simulink model "ORGANIZED_NominalTracking"  (R2024b)
settings: Solver=ode45  StartTime=0.0  StopTime=10  RelTol=1e-3
values from neighbouring files (symbols this model uses):
  current2Torque = mot.Kt    [simulation.m]
  denDriv = [Tdrv 1]    [simulation.m]
  denElect = [mot.L Req]    [simulation.m]
  denMech = [J_eq B_eq]    [simulation.m]
  numDriv = [kdrv]    [simulation.m]
  numElect = [1]    [simulation.m]
  numMech = [1]    [simulation.m]
  speed2Voltage = mot.Ke    [simulation.m]
undefined symbols (not defined in the file or in its folder): daq, degs2rpm, denBeam, denHPF, drv, gbox, kappa, mld, numBeam, numHPF, rads2rpm, rpm2rads, sens, ssc, ssc_LQR
settings Model: Creator=llp  LastModifiedBy=llp

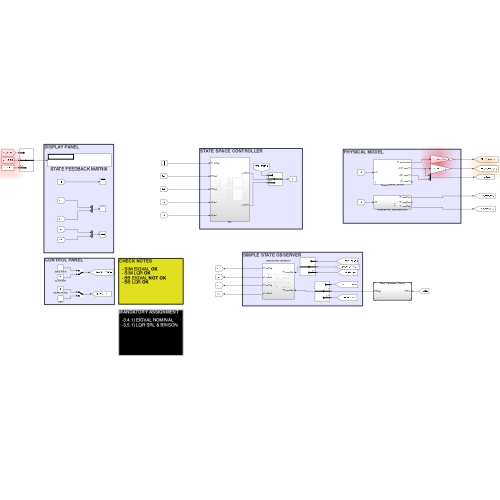
[thumbnail: Simulink's stored preview of the top-level diagram]
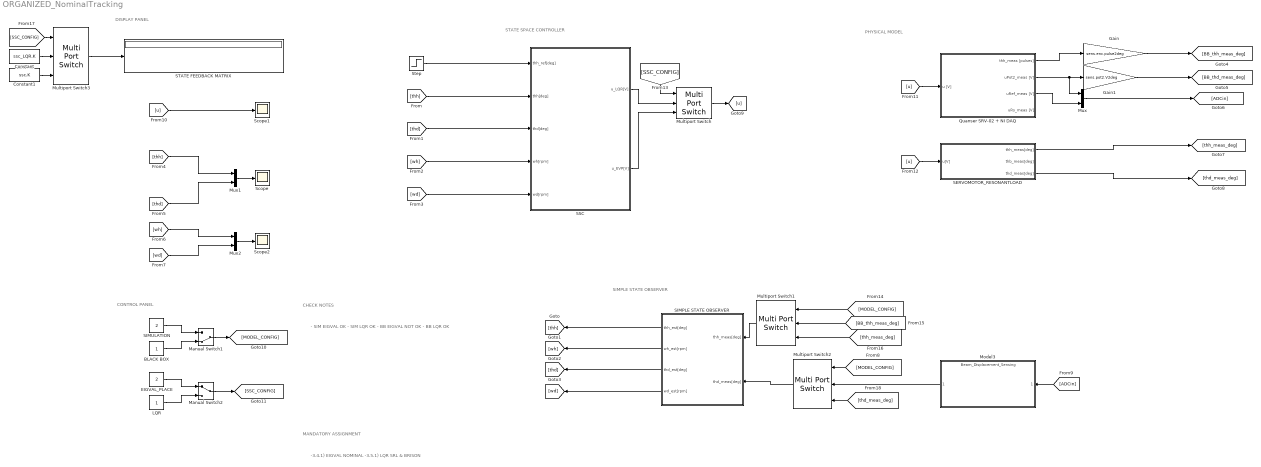
== system ORGANIZED_NominalTracking ==
  note: - SIM EIGVAL OK
      | - SIM LQR OK
      | - BB EIGVAL NOT OK
      | - BB LQR OK
  note: CHECK NOTES
  note: PHYSICAL MODEL
  note: STATE SPACE CONTROLLER
  note: SIMPLE STATE OBSERVER
  note: CONTROL PANEL
  note: DISPLAY PANEL
  note: -3.4.1) EIGVAL NOMINAL
      | -3.5.1) LQR SRL & BRISON
  note: MANDATORY ASSIGNMENT
  BLACK BOX : Constant
  Constant : Constant  Value=ssc_LQR.K
  Constant1 : Constant  Value=ssc.K
  EIGVAL_PLACE : Constant  Value=2
  Gain : Gain  Gain=sens.enc.pulse2deg
  Gain1 : Gain  Gain=sens.pot2.V2deg
  LQR : Constant
  Manual Switch1 : ManualSwitch  CurrentSetting=0
  Manual Switch2 : ManualSwitch
  Model3 : ModelReference  ModelNameDialog=Beam_Displacement_Sensing.slx  SimulationMode=Normal  ModelReferenceVersion=1.3
  Multiport Switch{,1..3} (4 alike) : MultiPortSwitch  Inputs=2  SaturateOnIntegerOverflow=off  InputSameDT=off
  Mux : Mux  Inputs=2
  Mux1 : Mux  Inputs=2
  Mux2 : Mux  Inputs=2
  Quanser SRV-02 + NI DAQ : Subsystem  mask(Quanser SRV-02 (with resonant load) + NI DAQ){Ts=0.001, fricType=Coulomb + viscous, lockShaft=off, beamInitPos=10}
      mask prompts: Ts "NI DAQ Sample Time:"; fricType "Friction model"; lockShaft "Lock motor shaft"; beamInitPos "Beam initial position [deg]:"
      mask help: Quanser SRV-02 (with resonant load) + NI DAQ model.
      mask init:
      | %%
      | % Riccardo Antonello (riccardo.antonello@unipd.it)
      | %
      | % April 28, 2020
      | %
      | % Dept. of Information Engineering, University of Padova
      | %
      | 
      | %%  Conversion gains
      | deg2rad = pi/180;                   %   [deg]   -> [rad]
      | rad2deg = 180/pi;                   %   [rad]   -> [deg]
      | 
      | 
      | %%  Sensors data
      | 
      | %   shunt resistor
      | sens.curr.Rs = 0.5;   
      | 
      | %   Hewlett-Packard HEDS-5540#A06 optical encoder
      | sens.enc.ppr = 500*4;                                                   %   pulses per rotation
      | sens.enc.pulse2deg = 360/sens.enc.ppr;                                  %   [pulses] -> [deg]
      | sens.enc.pulse2rad = 2*pi/sens.enc.ppr;                                 %   [pulses] -> [rad]
      | sens.enc.deg2pulse = sens.enc.ppr/360;                                  %   [deg] -> [pulses]
      | sens.enc.rad2pulse = sens.enc.ppr/2/pi;                                 %   [rad] -> [pulses]
      | 
      | %   potentiometer 2 (Spectrol 357-0-0-103) - installed on hub
      | sens.pot2.range.R      = 10e3;                                          %   ohmic value range 
      | sens.pot2.range.V      = 5;                                             %   voltage range
      | sens.pot2.range.th_deg = 340;                                           %   angle range [deg]
      | sens.pot2.range.th     = sens.pot2.range.th_deg * deg2rad;              %   angle range [rad]                           
      | sens.pot2.deg2V        = sens.pot2.range.V / sens.pot2.range.th_deg;    %   sensitivity [V/deg]
      | sens.pot2.rad2V        = sens.pot2.range.V / sens.pot2.range.th;        %   sensitivity [V/rad]
      | sens.pot2.V2deg        = 1/sens.pot2.deg2V;                             %   conversion gain [V] -> [deg]
      | sens.pot2.V2rad        = 1/sens.pot2.rad2V;                             %   conversion gain [V] -> [rad]
      | sens.pot2.noise.var    = 3.5e-7;                                        %   out noise variance [V^2]
      | 
      | 
      | %%  Data acquisition board (daq) data
      | 
      | %   NI PCI-6221 DAC data
      | daq.dac.bits = 16;                                  %   resolution (bits)
      | daq.dac.fs   = 10;                                  %   full scale 
      | daq.dac.q    = 2*daq.dac.fs/(2^daq.dac.bits-1);     %	quantization
      | 
      | %   NI PCI-6221 ADC data
      | daq.adc.bits = 16;                                  %   resolution (bits)
      | daq.adc.fs   = 10;                                  %   full scale (as set in SLDRT Analog Input block)
      | daq.adc.q    = 2*daq.adc.fs/(2^daq.adc.bits-1);     %   quantization   
      | 
      | 
      | %%  Set beam initial position
      | % SRV02Handle = find_system(gcb, ...
      | %     'LookUnderMasks', 'on', ...
      | %     'FindAll', 'on', ...
      | %     'FollowLinks', 'on', ...
      | %     'SearchDepth', '1', ...
      | %     'BlockType', 'ModelReference', ...
      | %     'Name', 'Quanser SRV-02');
      | %
      | % %get_param(SRV02Handle, 'InstanceParameters')
      | % InstanceParams = get_param(SRV02Handle, 'InstanceParameters');
      | % for k = 1:length(InstanceParams)
      | %     if strcmp(InstanceParams(k).Name, 'thb0')
      | %         if lockShaft
      | %             InstanceParams(k).Value = sprintf('%f', beamInitPos);
      | %         else
      | %             InstanceParams(k).Value = sprintf('%f', 0);    
      | %         end
      | %         set_param(SRV02Handle, 'InstanceParameters', InstanceParams);
      | %         break;
      | %     end
      | % end
      | 
      | if lockShaft
      |     thb0 = beamInitPos;
      | else
      |     thb0 = 0;    
      | end
      | 
      | 
      | %%  Mask initialization
      | if lockShaft
      |     
      |     %   find Inport handle
      |     InPortHandle = find_system(gcb, ...
      |         'LookUnderMasks', 'on', ...
      |         'FindAll', 'on', ...
      |         'FollowLinks', 'on', ...
      |         'SearchDepth', '1', ...
      |         'BlockType', 'Inport', ...
      |         'Name', 'u [V]');
      |     
      |     if ~isempty(InPortHandle)
      |     
      |         %   find DAC handle
      |         DACHandle = find_system(gcb, ...
      |             'LookUnderMasks', 'on', ...
      |             'FindAll', 'on', ...
      |             'FollowLinks', 'on', ...
      |             'SearchDepth', '1', ...
      |             'BlockType', 'SubSystem', ...
      |             'Name', 'DAC');  
      | 
      |         %   remove Inport output connection   
      |         InportConn = get_param(InPortHandle, 'PortConnectivity');
      |         delete_line(gcb, InportConn.Position);
      | 
      |         %   remove Inport block
      |         delete_block(InPortHandle);
      | 
      |         %   add Constant block
      |         ConstantHandle = add_block( ...
      |             'simulink/Sources/Constant', [gcb, '/u [V]'], ...
      |             'Position', [20   -37    50   -23], ...
      |             'Value', '0');
      | 
      |         %   connect Constant to DAC block
      |         DACPortHandles = get_param(DACHandle, 'PortHandles');
      |         ConstantPortHandles = get_param(ConstantHandle, 'PortHandles');
      |         add_line(gcb, ConstantPortHandles.Outport(1), DACPortHandles.Inport(1));
      |     
      |     end
      |     
      | else
      |     
      |     %   find Constant handle
      |     ConstantHandle = find_system(gcb, ...
      |         'LookUnderMasks', 'on', ...
      |         'FindAll', 'on', ...
      |         'FollowLinks', 'on', ...
      |         'SearchDepth', '1', ...
      |         'BlockType', 'Constant', ...
      |         'Name', 'u [V]');
      |     
      |     if ~isempty(ConstantHandle)
      |     
      |         %   find DAC handle
      |         DACHandle = find_system(gcb, ...
      |             'LookUnderMasks', 'on', ...
      |             'FindAll', 'on', ...
      |             'FollowLinks', 'on', ...
      |             'SearchDepth', '1', ...
      |             'BlockType', 'SubSystem', ...
      |             'Name', 'DAC');  
      |  
      |         %   remove Constant output connection   
      |         ConstantConn = get_param(ConstantHandle, 'PortConnectivity');
      |         delete_line(gcb, ConstantConn.Position);
      | 
      |         %   remove Inport block
      |         delete_block(ConstantHandle);   
      | 
      |         %   add Inport block
      |         InportHandle = add_block( ...
      |             'simulink/Sources/In1', [gcb, '/u [V]'], ...
      |             'Position', [20   -37    50   -23], ...
      |             'Port', '1');
      | 
      |         %   connect Constant to DAC block
      |         DACPortHandles = get_param(DACHandle, 'PortHandles');
      |         InportPortHandles = get_param(InportHandle, 'PortHandles');
      |         add_line(gcb, InportPortHandles.Outport(1), DACPortHandles.Inport(1));
      |     
      |      end
      |     
      | end
      mask Help:
      | Riccardo Antonello (antonello@dei.unipd.it)
      | 
      | April 28, 2020
      | 
      | Dept. of Information Engineering, University of Padova
      mask TypeOptions fricType: Coulomb + viscous | Karnopp
      mask Callback lockShaft:
      | %   get status of check box
      | lockShaft = get_param(gcb, 'lockShaft');
      | 
      | %   get current value of MaskVisibilities property
      | maskVisibilities = get_param(gcb, 'MaskVisibilities');
      | 
      | %   set visibility of the dialog box element
      | if strcmp(lockShaft, 'on')
      |     maskVisibilities{4} = 'on';
      | else
      |     maskVisibilities{4} = 'off';
      | end
      | 
      | % Set the 'MaskVisibilities' property for each parameter in mask
      | set_param( gcb, 'MaskVisibilities', maskVisibilities);
  SERVOMOTOR_RESONANTLOAD : Subsystem
  SIMPLE STATE OBSERVER : Subsystem
  SIMULATION : Constant  Value=2
  SSC : Subsystem
  STATE FEEDBACK MATRIX : Display
  Scope : Scope
  Scope1 : Scope
  Scope2 : Scope
  Step : Step  After=0  SampleTime=0
  wires:
  SIMPLE STATE OBSERVER/2(wh_est[rpm]) -> [wh]
  [thd] -> SSC/3(thd[deg])
  Gain/1 -> [BB_thh_meas_deg]
  Quanser SRV-02 + NI DAQ/2(uPot2_meas [V]) -> Mux/1, Gain1/1
  SIMPLE STATE OBSERVER/4(wd_est[rpm]) -> [wd]
  [wd] -> Mux2/2
  Mux1/1 -> Scope/1
  [wh] -> Mux2/1
  [thh] -> Mux1/1
  Quanser SRV-02 + NI DAQ/1(thh_meas [pulses]) -> Gain/1
  Mux2/1 -> Scope2/1
  Quanser SRV-02 + NI DAQ/3(uRef_meas [V]) -> Mux/2
  SIMPLE STATE OBSERVER/1(thh_est[deg]) -> [thh]
  SIMPLE STATE OBSERVER/3(thd_est[deg]) -> [thd]
  [thd] -> Mux1/2
  [thh] -> SSC/2(thh[deg])
  Gain1/1 -> [BB_thd_meas_deg]
  Mux/1 -> [ADCin]
  [ADCin] -> Model3/1
  SERVOMOTOR_RESONANTLOAD/3(thd_meas[deg]) -> [thd_meas_deg]
  SERVOMOTOR_RESONANTLOAD/1(thh_meas[deg]) -> [thh_meas_deg]
  Multiport Switch/1 -> [u]
  [u] -> Scope1/1
  [u] -> SERVOMOTOR_RESONANTLOAD/1(u[V])
  [wd] -> SSC/5(wd[rpm])
  [wh] -> SSC/4(wh[rpm])
  Step/1 -> SSC/1(thh_ref[deg])
  SSC/1(u_LQR[V]) -> Multiport Switch/2
  Manual Switch1/1 -> [MODEL_CONFIG]
  SIMULATION/1 -> Manual Switch1/1
  BLACK BOX/1 -> Manual Switch1/2
  LQR/1 -> Manual Switch2/2
  Manual Switch2/1 -> [SSC_CONFIG]
  EIGVAL_PLACE/1 -> Manual Switch2/1
  [SSC_CONFIG] -> Multiport Switch/1
  SSC/2(u_EVP[V]) -> Multiport Switch/3
  [MODEL_CONFIG] -> Multiport Switch1/1
  [BB_thh_meas_deg] -> Multiport Switch1/2
  [thh_meas_deg] -> Multiport Switch1/3
  [MODEL_CONFIG] -> Multiport Switch2/1
  Model3/1 -> Multiport Switch2/2
  [thd_meas_deg] -> Multiport Switch2/3
  Multiport Switch2/1 -> SIMPLE STATE OBSERVER/2(thd_meas[deg])
  Multiport Switch1/1 -> SIMPLE STATE OBSERVER/1(thh_meas[deg])
  [SSC_CONFIG] -> Multiport Switch3/1
  Constant/1 -> Multiport Switch3/2
  Constant1/1 -> Multiport Switch3/3
  Multiport Switch3/1 -> STATE FEEDBACK MATRIX/1
  [u] -> Quanser SRV-02 + NI DAQ/1(u [V])

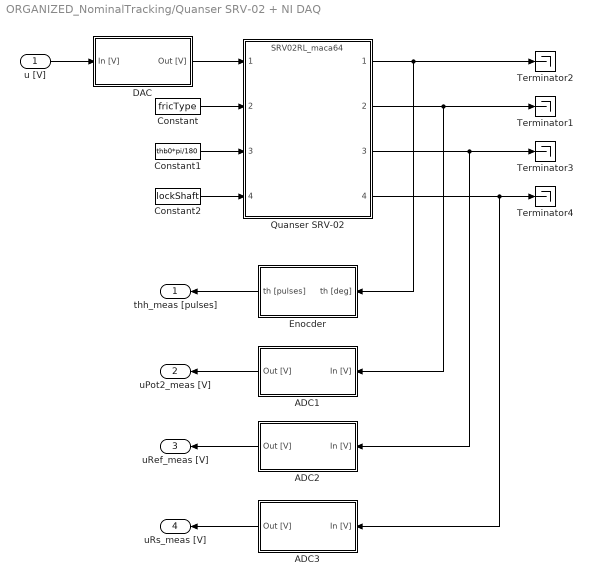
== system ORGANIZED_NominalTracking/Quanser SRV-02 + NI DAQ ==
  u [V] : Inport
  ADC1 : Subsystem
  ADC2 : Subsystem
  ADC3 : Subsystem
  Constant : Constant  Value=fricType
  Constant1 : Constant  Value=thb0*pi/180  SampleTime=Inf
  Constant2 : Constant  Value=lockShaft  SampleTime=Inf
  DAC : Subsystem
  Enocder : Subsystem
  Quanser SRV-02 : ModelReference  ModelNameDialog=SRV02RL_maca64.slxp  ModelReferenceVersion=1.76  CopyOfModelProtected=on
  Terminator{1..4} (4 alike) : Terminator
  thh_meas [pulses] : Outport
  uPot2_meas [V] : Outport  Port=2
  uRef_meas [V] : Outport  Port=3
  uRs_meas [V] : Outport  Port=4
  wires:
  Enocder/1(th [pulses]) -> thh_meas [pulses]/1
  ADC3/1(Out [V]) -> uRs_meas [V]/1
  DAC/1(Out [V]) -> Quanser SRV-02/1
  Quanser SRV-02/2 -> ADC1/1(In [V]), Terminator1/1
  Quanser SRV-02/1 -> Terminator2/1, Enocder/1(th [deg])
  Constant/1 -> Quanser SRV-02/2
  Quanser SRV-02/3 -> ADC2/1(In [V]), Terminator3/1
  ADC1/1(Out [V]) -> uPot2_meas [V]/1
  Constant1/1 -> Quanser SRV-02/3
  Constant2/1 -> Quanser SRV-02/4
  Quanser SRV-02/4 -> ADC3/1(In [V]), Terminator4/1
  ADC2/1(Out [V]) -> uRef_meas [V]/1
  u [V]/1 -> DAC/1(In [V])

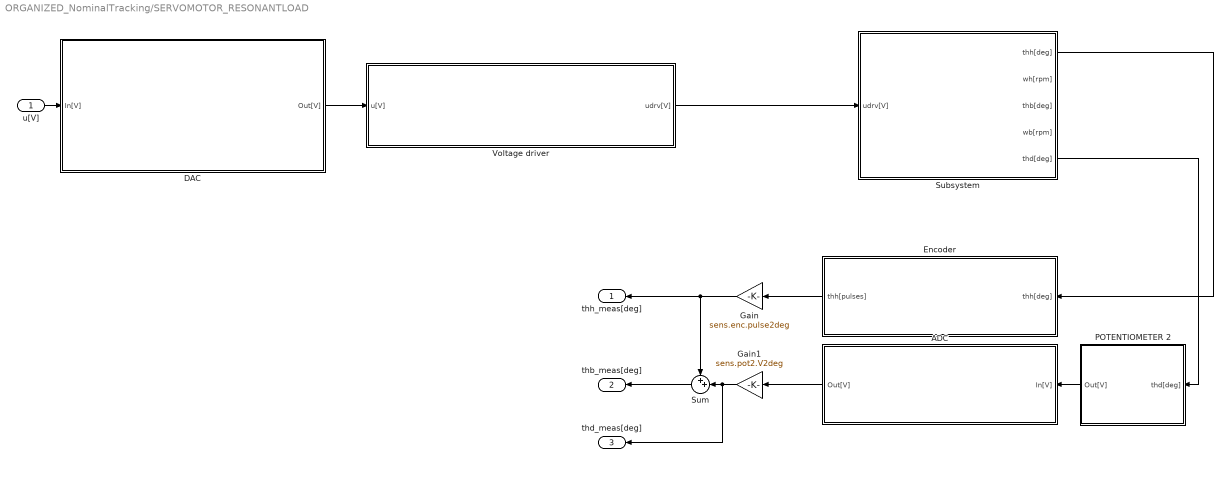
== system ORGANIZED_NominalTracking/SERVOMOTOR_RESONANTLOAD ==
  u[V] : Inport
  ADC : Subsystem
  DAC : Subsystem
  Encoder : Subsystem
  Gain : Gain  Gain=sens.enc.pulse2deg
  Gain1 : Gain  Gain=sens.pot2.V2deg
  POTENTIOMETER 2 : Subsystem
  Subsystem : Subsystem
  Sum : Sum  Inputs=++|
  Voltage driver : Subsystem
  thh_meas[deg] : Outport
  thb_meas[deg] : Outport  Port=2
  thd_meas[deg] : Outport  Port=3
  wires:
  Sum/1 -> thb_meas[deg]/1
  POTENTIOMETER 2/1(Out[V]) -> ADC/1(In[V])
  Gain/1 -> Sum/1, thh_meas[deg]/1
  ADC/1(Out[V]) -> Gain1/1
  u[V]/1 -> DAC/1(In[V])
  Encoder/1(thh[pulses]) -> Gain/1
  Subsystem/1(thh[deg]) -> Encoder/1(thh[deg])
  Voltage driver/1(udrv[V]) -> Subsystem/1(udrv[V])
  DAC/1(Out[V]) -> Voltage driver/1(u[V])
  Subsystem/5(thd[deg]) -> POTENTIOMETER 2/1(thd[deg])
  Gain1/1 -> thd_meas[deg]/1, Sum/2

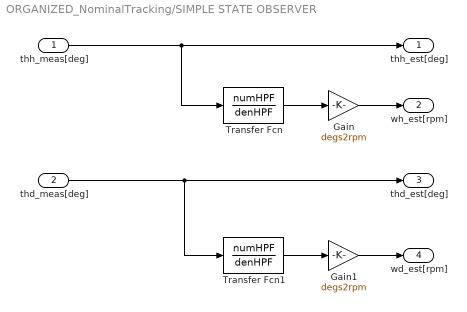
== system ORGANIZED_NominalTracking/SIMPLE STATE OBSERVER ==
  thh_meas[deg] : Inport
  thd_meas[deg] : Inport  Port=2
  Gain : Gain  Gain=degs2rpm
  Gain1 : Gain  Gain=degs2rpm
  Transfer Fcn : TransferFcn  Numerator=numHPF  Denominator=denHPF
  Transfer Fcn1 : TransferFcn  Numerator=numHPF  Denominator=denHPF
  thh_est[deg] : Outport
  wh_est[rpm] : Outport  Port=2
  thd_est[deg] : Outport  Port=3
  wd_est[rpm] : Outport  Port=4
  wires:
  thh_meas[deg]/1 -> Transfer Fcn/1, thh_est[deg]/1
  Gain1/1 -> wd_est[rpm]/1
  thd_meas[deg]/1 -> Transfer Fcn1/1, thd_est[deg]/1
  Transfer Fcn1/1 -> Gain1/1
  Transfer Fcn/1 -> Gain/1
  Gain/1 -> wh_est[rpm]/1

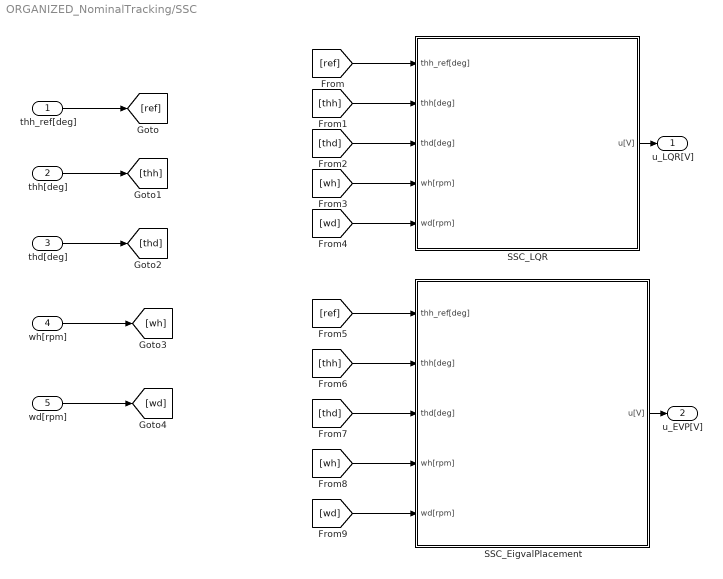
== system ORGANIZED_NominalTracking/SSC ==
  thh_ref[deg] : Inport
  thh[deg] : Inport  Port=2
  thd[deg] : Inport  Port=3
  wh[rpm] : Inport  Port=4
  wd[rpm] : Inport  Port=5
  SSC_EigvalPlacement : Subsystem
  SSC_LQR : Subsystem
  u_LQR[V] : Outport
  u_EVP[V] : Outport  Port=2
  wires:
  SSC_EigvalPlacement/1(u[V]) -> u_EVP[V]/1
  SSC_LQR/1(u[V]) -> u_LQR[V]/1
  wd[rpm]/1 -> [wd]
  wh[rpm]/1 -> [wh]
  thd[deg]/1 -> [thd]
  thh[deg]/1 -> [thh]
  thh_ref[deg]/1 -> [ref]
  [ref] -> SSC_LQR/1(thh_ref[deg])
  [thh] -> SSC_LQR/2(thh[deg])
  [thd] -> SSC_LQR/3(thd[deg])
  [wh] -> SSC_LQR/4(wh[rpm])
  [wd] -> SSC_LQR/5(wd[rpm])
  [ref] -> SSC_EigvalPlacement/1(thh_ref[deg])
  [thh] -> SSC_EigvalPlacement/2(thh[deg])
  [thd] -> SSC_EigvalPlacement/3(thd[deg])
  [wh] -> SSC_EigvalPlacement/4(wh[rpm])
  [wd] -> SSC_EigvalPlacement/5(wd[rpm])

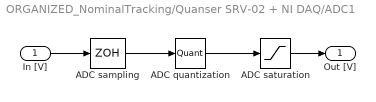
== system ORGANIZED_NominalTracking/Quanser SRV-02 + NI DAQ/ADC1 ==
  In [V] : Inport
  ADC quantization : Quantizer  QuantizationInterval=daq.adc.q
  ADC sampling : ZeroOrderHold  SampleTime=Ts
  ADC saturation : Saturate  UpperLimit=daq.adc.fs  LowerLimit=-daq.adc.fs
  Out [V] : Outport
  wires:
  ADC saturation/1 -> Out [V]/1
  ADC sampling/1 -> ADC quantization/1
  In [V]/1 -> ADC sampling/1
  ADC quantization/1 -> ADC saturation/1

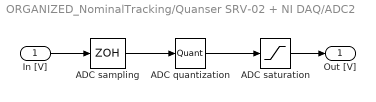
== system ORGANIZED_NominalTracking/Quanser SRV-02 + NI DAQ/ADC2 ==
  In [V] : Inport
  ADC quantization : Quantizer  QuantizationInterval=daq.adc.q
  ADC sampling : ZeroOrderHold  SampleTime=Ts
  ADC saturation : Saturate  UpperLimit=daq.adc.fs  LowerLimit=-daq.adc.fs
  Out [V] : Outport
  wires:
  ADC quantization/1 -> ADC saturation/1
  In [V]/1 -> ADC sampling/1
  ADC sampling/1 -> ADC quantization/1
  ADC saturation/1 -> Out [V]/1

== system ORGANIZED_NominalTracking/Quanser SRV-02 + NI DAQ/ADC3 ==
  In [V] : Inport
  Quantizer : Quantizer  QuantizationInterval=daq.adc.q
  Saturation : Saturate  UpperLimit=daq.adc.fs  LowerLimit=-daq.adc.fs
  Zero-Order Hold : ZeroOrderHold  SampleTime=Ts
  Out [V] : Outport
  wires:
  Saturation/1 -> Out [V]/1
  In [V]/1 -> Zero-Order Hold/1
  Quantizer/1 -> Saturation/1
  Zero-Order Hold/1 -> Quantizer/1

== system ORGANIZED_NominalTracking/Quanser SRV-02 + NI DAQ/DAC ==
  In [V] : Inport
  Quantizer : Quantizer  QuantizationInterval=daq.dac.q
  Saturation : Saturate  UpperLimit=daq.dac.fs  LowerLimit=-daq.dac.fs
  Zero-Order Hold : ZeroOrderHold  SampleTime=Ts
  Out [V] : Outport
  wires:
  Quantizer/1 -> Saturation/1
  In [V]/1 -> Zero-Order Hold/1
  Zero-Order Hold/1 -> Quantizer/1
  Saturation/1 -> Out [V]/1

== system ORGANIZED_NominalTracking/Quanser SRV-02 + NI DAQ/Enocder ==
  th [deg] : Inport
  Quantizer : Quantizer  QuantizationInterval=sens.enc.pulse2deg
  Zero-Order Hold : ZeroOrderHold  SampleTime=Ts
  deg2pulse : Gain  Gain=sens.enc.deg2pulse
  th [pulses] : Outport
  wires:
  Quantizer/1 -> deg2pulse/1
  th [deg]/1 -> Zero-Order Hold/1
  Zero-Order Hold/1 -> Quantizer/1
  deg2pulse/1 -> th [pulses]/1

== system ORGANIZED_NominalTracking/SERVOMOTOR_RESONANTLOAD/ADC ==
  In[V] : Inport
  Quantizer : Quantizer  QuantizationInterval=daq.adc.q
  Saturation : Saturate  UpperLimit=daq.adc.fs  LowerLimit=-daq.adc.fs
  Zero-Order Hold : ZeroOrderHold  SampleTime=daq.adc.ts
  Out[V] : Outport
  wires:
  Saturation/1 -> Out[V]/1
  In[V]/1 -> Zero-Order Hold/1
  Zero-Order Hold/1 -> Quantizer/1
  Quantizer/1 -> Saturation/1

== system ORGANIZED_NominalTracking/SERVOMOTOR_RESONANTLOAD/DAC ==
  In[V] : Inport
  Quantizer : Quantizer  QuantizationInterval=daq.dac.q
  Saturation : Saturate  UpperLimit=daq.dac.fs  LowerLimit=-daq.dac.fs
  Zero-Order Hold : ZeroOrderHold  SampleTime=daq.dac.ts
  Out[V] : Outport
  wires:
  Saturation/1 -> Out[V]/1
  In[V]/1 -> Zero-Order Hold/1
  Zero-Order Hold/1 -> Quantizer/1
  Quantizer/1 -> Saturation/1

== system ORGANIZED_NominalTracking/SERVOMOTOR_RESONANTLOAD/Encoder ==
  thh[deg] : Inport
  Gain : Gain  Gain=sens.enc.deg2pulse
  Quantizer : Quantizer  QuantizationInterval=daq.adc.q
  Zero-Order Hold : ZeroOrderHold  SampleTime=daq.adc.ts
  thh[pulses] : Outport
  wires:
  thh[deg]/1 -> Zero-Order Hold/1
  Gain/1 -> thh[pulses]/1
  Quantizer/1 -> Gain/1
  Zero-Order Hold/1 -> Quantizer/1

== system ORGANIZED_NominalTracking/SERVOMOTOR_RESONANTLOAD/POTENTIOMETER 2 ==
  thd[deg] : Inport
  Gain2 : Gain  Gain=sens.pot2.deg2V
  Random Number : RandomNumber  Variance=sens.pot2.noise.var  SampleTime=sens.pot2.Ts
  Sum1 : Sum  Inputs=++|
  Out[V] : Outport
  wires:
  thd[deg]/1 -> Gain2/1
  Gain2/1 -> Sum1/2
  Random Number/1 -> Sum1/1
  Sum1/1 -> Out[V]/1

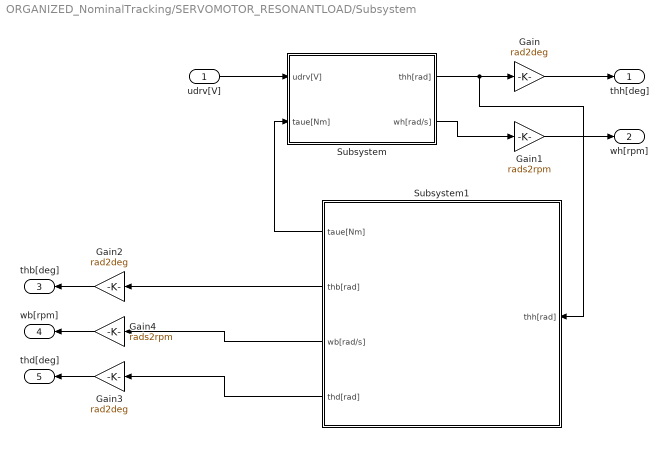
== system ORGANIZED_NominalTracking/SERVOMOTOR_RESONANTLOAD/Subsystem ==
  udrv[V] : Inport
  Gain : Gain  Gain=rad2deg
  Gain1 : Gain  Gain=rads2rpm
  Gain2 : Gain  Gain=rad2deg
  Gain3 : Gain  Gain=rad2deg
  Gain4 : Gain  Gain=rads2rpm
  Subsystem : Subsystem
  Subsystem1 : Subsystem
  thh[deg] : Outport
  wh[rpm] : Outport  Port=2
  thb[deg] : Outport  Port=3
  wb[rpm] : Outport  Port=4
  thd[deg] : Outport  Port=5
  wires:
  Subsystem1/1(taue[Nm]) -> Subsystem/2(taue[Nm])
  Gain1/1 -> wh[rpm]/1
  Gain2/1 -> thb[deg]/1
  Subsystem1/2(thb[rad]) -> Gain2/1
  Gain/1 -> thh[deg]/1
  Gain4/1 -> wb[rpm]/1
  Gain3/1 -> thd[deg]/1
  Subsystem/2(wh[rad/s]) -> Gain1/1
  udrv[V]/1 -> Subsystem/1(udrv[V])
  Subsystem/1(thh[rad]) -> Subsystem1/1(thh[rad]), Gain/1
  Subsystem1/4(thd[rad]) -> Gain3/1
  Subsystem1/3(wb[rad/s]) -> Gain4/1

== system ORGANIZED_NominalTracking/SERVOMOTOR_RESONANTLOAD/Voltage driver ==
  u[V] : Inport
  Saturation : Saturate  UpperLimit=drv.outmax  LowerLimit=-drv.outmax
  Transfer Fcn1 : TransferFcn  Numerator=numDriv  Denominator=denDriv
  udrv[V] : Outport
  wires:
  u[V]/1 -> Transfer Fcn1/1
  Saturation/1 -> udrv[V]/1
  Transfer Fcn1/1 -> Saturation/1

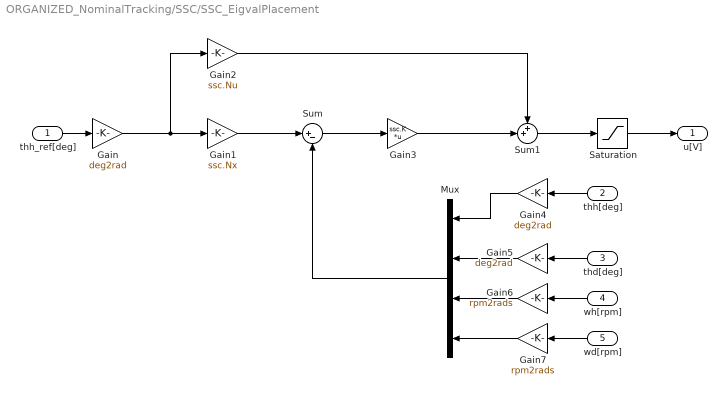
== system ORGANIZED_NominalTracking/SSC/SSC_EigvalPlacement ==
  thh_ref[deg] : Inport
  thh[deg] : Inport  Port=2
  thd[deg] : Inport  Port=3
  wh[rpm] : Inport  Port=4
  wd[rpm] : Inport  Port=5
  Gain : Gain  Gain=deg2rad
  Gain1 : Gain  Gain=ssc.Nx
  Gain2 : Gain  Gain=ssc.Nu
  Gain3 : Gain  Gain=ssc.K  Multiplication=Matrix(K*u)
  Gain4 : Gain  Gain=deg2rad
  Gain5 : Gain  Gain=deg2rad
  Gain6 : Gain  Gain=rpm2rads
  Gain7 : Gain  Gain=rpm2rads
  Mux : Mux
  Saturation : Saturate  UpperLimit=drv.outmax  LowerLimit=-drv.outmax
  Sum : Sum  Inputs=|+-
  Sum1 : Sum  Inputs=++|
  u[V] : Outport
  wires:
  Gain1/1 -> Sum/1
  thh[deg]/1 -> Gain4/1
  Saturation/1 -> u[V]/1
  wh[rpm]/1 -> Gain6/1
  Gain/1 -> Gain2/1, Gain1/1
  thh_ref[deg]/1 -> Gain/1
  Gain4/1 -> Mux/1
  Sum1/1 -> Saturation/1
  thd[deg]/1 -> Gain5/1
  Gain6/1 -> Mux/3
  Gain5/1 -> Mux/2
  Gain2/1 -> Sum1/1
  Sum/1 -> Gain3/1
  Gain3/1 -> Sum1/2
  Gain7/1 -> Mux/4
  wd[rpm]/1 -> Gain7/1
  Mux/1 -> Sum/2

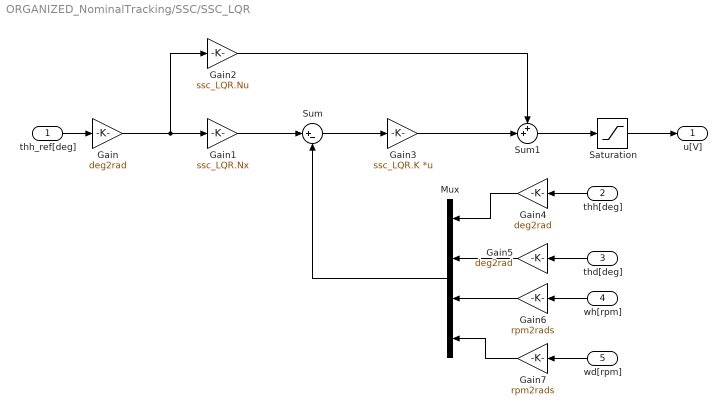
== system ORGANIZED_NominalTracking/SSC/SSC_LQR ==
  thh_ref[deg] : Inport
  thh[deg] : Inport  Port=2
  thd[deg] : Inport  Port=3
  wh[rpm] : Inport  Port=4
  wd[rpm] : Inport  Port=5
  Gain : Gain  Gain=deg2rad
  Gain1 : Gain  Gain=ssc_LQR.Nx
  Gain2 : Gain  Gain=ssc_LQR.Nu
  Gain3 : Gain  Gain=ssc_LQR.K  Multiplication=Matrix(K*u)
  Gain4 : Gain  Gain=deg2rad
  Gain5 : Gain  Gain=deg2rad
  Gain6 : Gain  Gain=rpm2rads
  Gain7 : Gain  Gain=rpm2rads
  Mux : Mux
  Saturation : Saturate  UpperLimit=drv.outmax  LowerLimit=-drv.outmax
  Sum : Sum  Inputs=|+-
  Sum1 : Sum  Inputs=++|
  u[V] : Outport
  wires:
  Sum/1 -> Gain3/1
  wd[rpm]/1 -> Gain7/1
  Gain6/1 -> Mux/3
  wh[rpm]/1 -> Gain6/1
  thh[deg]/1 -> Gain4/1
  Gain7/1 -> Mux/4
  thh_ref[deg]/1 -> Gain/1
  Sum1/1 -> Saturation/1
  Gain3/1 -> Sum1/2
  thd[deg]/1 -> Gain5/1
  Gain/1 -> Gain2/1, Gain1/1
  Gain5/1 -> Mux/2
  Mux/1 -> Sum/2
  Gain2/1 -> Sum1/1
  Gain1/1 -> Sum/1
  Gain4/1 -> Mux/1
  Saturation/1 -> u[V]/1

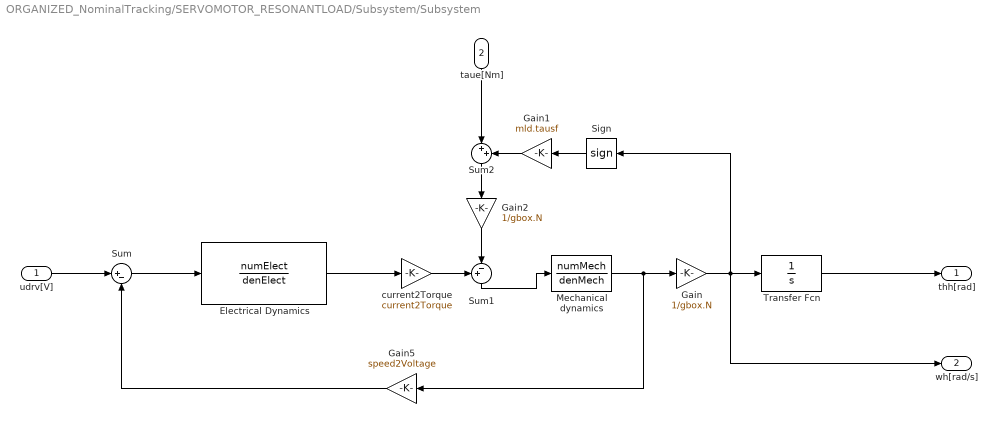
== system ORGANIZED_NominalTracking/SERVOMOTOR_RESONANTLOAD/Subsystem/Subsystem ==
  udrv[V] : Inport
  taue[Nm] : Inport  Port=2
  " Electrical Dynamics" : TransferFcn  Numerator=numElect  Denominator=denElect
  Gain : Gain  Gain=1/gbox.N
  Gain1 : Gain  Gain=mld.tausf
  Gain2 : Gain  Gain=1/gbox.N
  Gain5 : Gain  Gain=speed2Voltage
  Mechanical dynamics : TransferFcn  Numerator=numMech  Denominator=denMech
  Sign : Signum  ZeroCross=off
  Sum : Sum  Inputs=|+-
  Sum1 : Sum  Inputs=+-|
  Sum2 : Sum  Inputs=|++
  Transfer Fcn : TransferFcn  Denominator=[1 0]
  current2Torque : Gain  Gain=current2Torque
  thh[rad] : Outport
  wh[rad/s] : Outport  Port=2
  wires:
  Transfer Fcn/1 -> thh[rad]/1
  Gain/1 -> wh[rad/s]/1, Transfer Fcn/1, Sign/1
  udrv[V]/1 -> Sum/1
  Mechanical dynamics/1 -> Gain5/1, Gain/1
  current2Torque/1 -> Sum1/1
  Sum2/1 -> Gain2/1
  Gain2/1 -> Sum1/2
  taue[Nm]/1 -> Sum2/1
  " Electrical Dynamics"/1 -> current2Torque/1
  Gain1/1 -> Sum2/2
  Sign/1 -> Gain1/1
  Gain5/1 -> Sum/2
  Sum/1 -> " Electrical Dynamics"/1
  Sum1/1 -> Mechanical dynamics/1

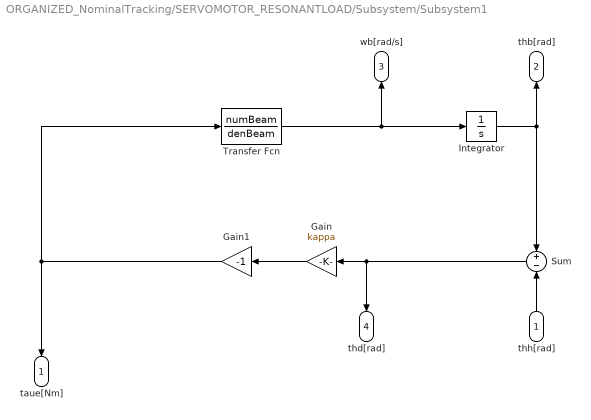
== system ORGANIZED_NominalTracking/SERVOMOTOR_RESONANTLOAD/Subsystem/Subsystem1 ==
  thh[rad] : Inport
  Gain : Gain  Gain=kappa
  Gain1 : Gain  Gain=-1
  Integrator : Integrator
  Sum : Sum  Inputs=+-
  Transfer Fcn : TransferFcn  Numerator=numBeam  Denominator=denBeam
  taue[Nm] : Outport
  thb[rad] : Outport  Port=2
  wb[rad/s] : Outport  Port=3
  thd[rad] : Outport  Port=4
  wires:
  Integrator/1 -> Sum/1, thb[rad]/1
  Gain/1 -> Gain1/1
  thh[rad]/1 -> Sum/2
  Transfer Fcn/1 -> Integrator/1, wb[rad/s]/1
  Gain1/1 -> taue[Nm]/1, Transfer Fcn/1
  Sum/1 -> Gain/1, thd[rad]/1
